simulink model "solow_simulink"  (R2025b)
settings: Solver=VariableStepAuto  StartTime=0.0  StopTime=200  RelTol=1e-3
values from neighbouring files (symbols this model uses):
  A = params.A    [solow_ode.m]    (also in solow_params.m = 1)
  alpha = params.alpha    [solow_ode.m]    (also in solow_params.m = 0.33)
  delta = params.delta    [solow_ode.m]    (also in solow_params.m = 0.05)
  k0 = 0.1    [run_solow.m]    (also in solow_params.m)
  n = params.n    [solow_ode.m]    (also in solow_params.m = 0.02)
  s = params.s    [solow_ode.m]    (also in solow_params.m = 0.25)

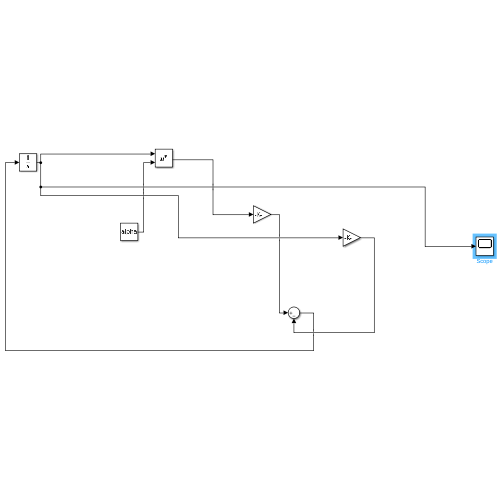
[thumbnail: Simulink's stored preview of the top-level diagram]
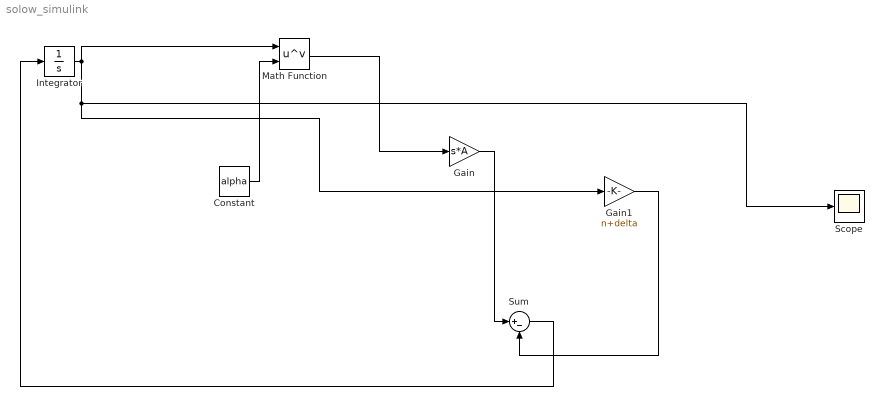
== system solow_simulink ==
  Constant : Constant  Value=alpha
  Gain : Gain  Gain=s*A
  Gain1 : Gain  Gain=n+delta
  Integrator : Integrator  InitialCondition=k0
  Math Function : Math  Operator=pow
  Scope : Scope
      settings: ActiveDisplayYMinimum=-0.72309502820469618  ActiveDisplayYMaximum=7.5078552538422683
  Sum : Sum  Inputs=|+-
  wires:
  Constant/1 -> Math Function/2
  Integrator/1 -> Scope/1, Gain1/1, Math Function/1
  Math Function/1 -> Gain/1
  Gain1/1 -> Sum/2
  Gain/1 -> Sum/1
  Sum/1 -> Integrator/1
